simulink model "GeschlossenerKreis"  (R2017b)
settings: Solver=VariableStepAuto  StartTime=0.0  StopTime=0.1  RelTol=1e-3
libraries: cstblocks x4, simulink x1
settings Model: Creator=user  LastModifiedBy=user
settings SFSimCC: SimUseLocalCustomCode=on
settings RTWCC: RTWUseLocalCustomCode=on

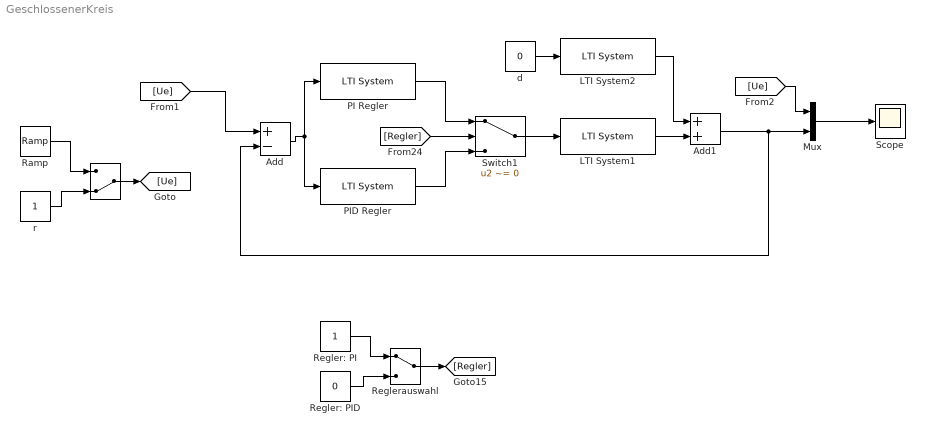
== system GeschlossenerKreis ==
  " " : ManualSwitch  CurrentSetting=0
  Add : Sum  Inputs=+-
  Add1 : Sum
  LTI System1 : cstblocks/LTI System  sys=G  IC=[]
  LTI System2 : cstblocks/LTI System  sys=Gd  IC=[]
  Mux : Mux  Inputs=2
  PI Regler : cstblocks/LTI System  sys=R_pi  IC=[]
  PID Regler : cstblocks/LTI System  sys=R_pid  IC=[]
  Ramp : simulink/Sources/Ramp  slope=1  start=0  X0=0
  Regler: PI : Constant
  Regler: PID : Constant  Value=0
  Reglerauswahl : ManualSwitch
  Scope : Scope
  Switch1 : Switch  Criteria=u2 ~= 0
  d : Constant  Value=0
  r : Constant
  wires:
  [Ue] -> Mux/1
  [Regler] -> Switch1/2
  Regler: PI/1 -> Reglerauswahl/1
  LTI System1/1 -> Add1/2
  r/1 -> " "/2
  Reglerauswahl/1 -> [Regler]
  " "/1 -> [Ue]
  LTI System2/1 -> Add1/1
  [Ue] -> Add/1
  d/1 -> LTI System2/1
  Mux/1 -> Scope/1
  PI Regler/1 -> Switch1/1
  Add1/1 -> Add/2, Mux/2
  Ramp/1 -> " "/1
  Regler: PID/1 -> Reglerauswahl/2
  Add/1 -> PID Regler/1, PI Regler/1
  PID Regler/1 -> Switch1/3
  Switch1/1 -> LTI System1/1
